simulink library "v2l"  (R2021b)
settings: Solver=VariableStepAuto  StartTime=0.0  StopTime=10.0  RelTol=1e-3
undefined symbols (not defined in the file or in its folder): KV2L_HVBattSOCLimit_pct, KV2L_SOCV2LSetLimit_pct
libraries: nmm x1, FVT_lib x1
settings Model: Creator=FVT23010  LastModifiedBy=FVT23010

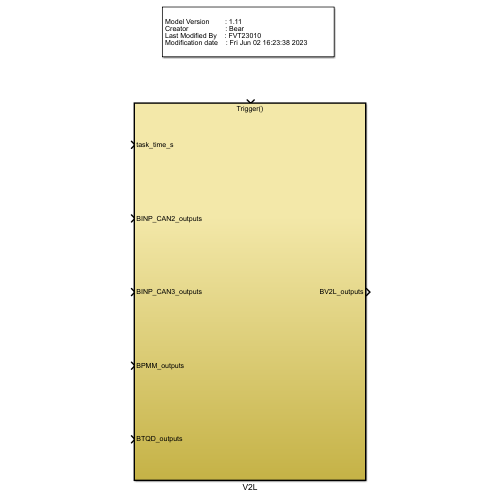
[thumbnail: Simulink's stored preview of the top-level diagram]
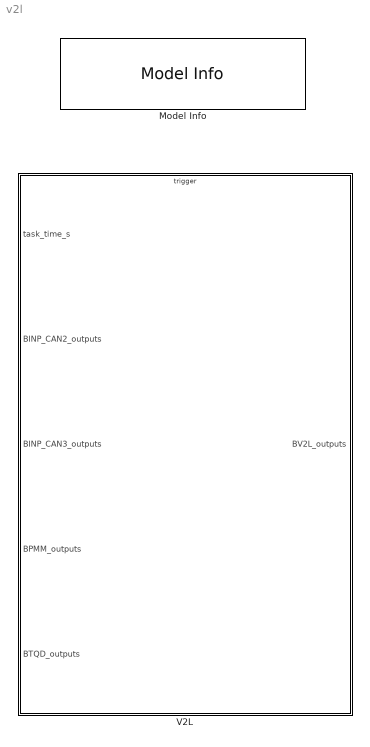
== system v2l ==
  Model Info : nmm/Model Info  InitialBlockCM=None  BlockCM=None  Frame=on  DisplayStringWithTags=|  HorizontalTextAlignment=Left  LeftAlignmentValue=0.02  SourceBlockDiagram=pmm  TagMaxNumber=20
      | Model Version        : %<ModelVersion>
      | Creator                   : Bear
      | Last Modified By    : %<LastModifiedBy>
      | Modification date    : %<LastModificationDate>
  V2L : Subsystem
      settings: RTWSystemCode=Nonreusable function  RTWFcnNameOpts=Use subsystem name  RTWFileNameOpts=Use subsystem name

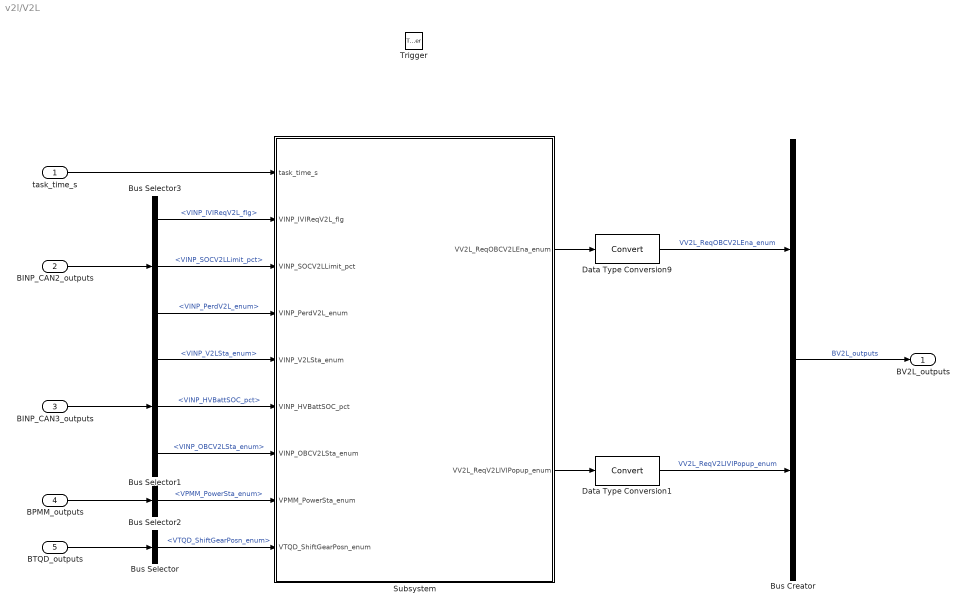
== system v2l/V2L ==
  task_time_s : Inport
  BINP_CAN2_outputs : Inport  Port=2  OutDataTypeStr=Bus: BINP_CAN2_outputs
  BINP_CAN3_outputs : Inport  Port=3  OutDataTypeStr=Bus: BINP_CAN3_outputs
  BPMM_outputs : Inport  Port=4  OutDataTypeStr=Bus: BPMM_outputs
  BTQD_outputs : Inport  Port=5  OutDataTypeStr=Bus: BTQD_outputs
  Trigger : TriggerPort  TriggerType=function-call  VariantControl=(inherit)  PortDimensions=1
  Bus Creator : BusCreator  Inputs=2  OutDataTypeStr=Bus: BV2L_outputs
  Bus Selector : BusSelector  OutputSignals=VTQD_ShiftGearPosn_enum
  Bus Selector1 : BusSelector  OutputSignals=VINP_V2LSta_enum,VINP_HVBattSOC_pct,VINP_OBCV2LSta_enum
  Bus Selector2 : BusSelector  OutputSignals=VPMM_PowerSta_enum
  Bus Selector3 : BusSelector  OutputSignals=VINP_IVIReqV2L_flg,VINP_SOCV2LLimit_pct,VINP_PerdV2L_enum
  Data Type Conversion1 : DataTypeConversion
  Data Type Conversion9 : DataTypeConversion
  Subsystem : Subsystem
  BV2L_outputs : Outport  OutDataTypeStr=Bus: BV2L_outputs
  wires:
  Bus Creator/1 -> BV2L_outputs/1  "BV2L_outputs"
  Subsystem/1(VV2L_ReqOBCV2LEna_enum) -> Data Type Conversion9/1
  Subsystem/2(VV2L_ReqV2LIVIPopup_enum) -> Data Type Conversion1/1
  task_time_s/1 -> Subsystem/1(task_time_s)
  BTQD_outputs/1 -> Bus Selector/1
  Bus Selector/1 -> Subsystem/9(VTQD_ShiftGearPosn_enum)  "<VTQD_ShiftGearPosn_enum>"
  BINP_CAN3_outputs/1 -> Bus Selector1/1
  Bus Selector1/2 -> Subsystem/6(VINP_HVBattSOC_pct)  "<VINP_HVBattSOC_pct>"
  BPMM_outputs/1 -> Bus Selector2/1
  Bus Selector2/1 -> Subsystem/8(VPMM_PowerSta_enum)  "<VPMM_PowerSta_enum>"
  BINP_CAN2_outputs/1 -> Bus Selector3/1
  Bus Selector3/2 -> Subsystem/3(VINP_SOCV2LLimit_pct)  "<VINP_SOCV2LLimit_pct>"
  Bus Selector3/1 -> Subsystem/2(VINP_IVIReqV2L_flg)  "<VINP_IVIReqV2L_flg>"
  Bus Selector3/3 -> Subsystem/4(VINP_PerdV2L_enum)  "<VINP_PerdV2L_enum>"
  Bus Selector1/1 -> Subsystem/5(VINP_V2LSta_enum)  "<VINP_V2LSta_enum>"
  Bus Selector1/3 -> Subsystem/7(VINP_OBCV2LSta_enum)  "<VINP_OBCV2LSta_enum>"
  Data Type Conversion9/1 -> Bus Creator/1  "VV2L_ReqOBCV2LEna_enum"
  Data Type Conversion1/1 -> Bus Creator/2  "VV2L_ReqV2LIVIPopup_enum"

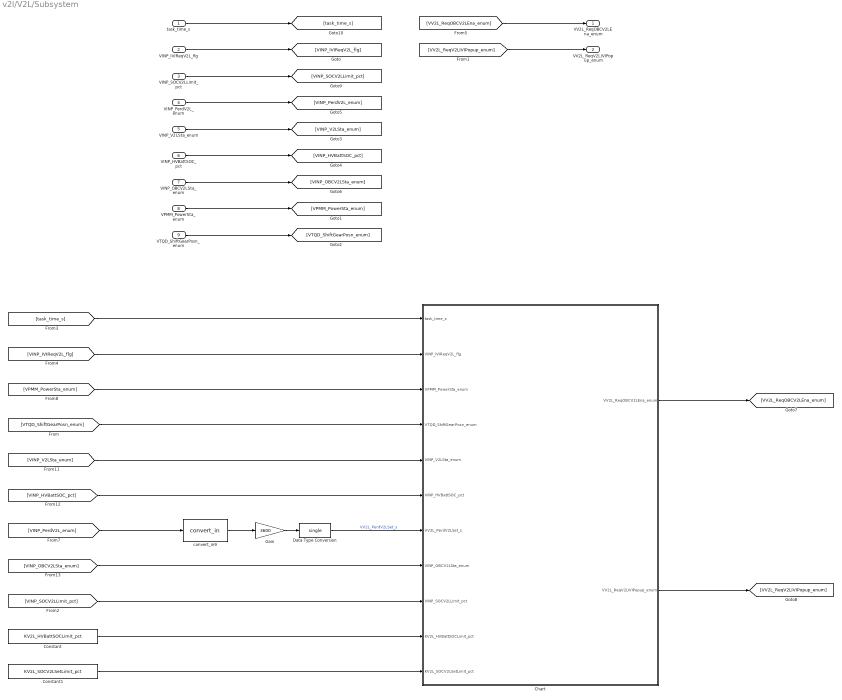
== system v2l/V2L/Subsystem ==
  task_time_s : Inport
  VINP_IVIReqV2L_flg : Inport  Port=2
  VINP_SOCV2LLimit_pct : Inport  Port=3
  VINP_PerdV2L_enum : Inport  Port=4
  VINP_V2LSta_enum : Inport  Port=5
  VINP_HVBattSOC_pct : Inport  Port=6
  VINP_OBCV2LSta_enum : Inport  Port=7
  VPMM_PowerSta_enum : Inport  Port=8
  VTQD_ShiftGearPosn_enum : Inport  Port=9
  Chart : Stateflow chart  TreatAsAtomicUnit=on
  Constant : Constant  Value=KV2L_HVBattSOCLimit_pct
  Constant1 : Constant  Value=KV2L_SOCV2LSetLimit_pct
  Data Type Conversion : DataTypeConversion  OutDataTypeStr=single
  Gain : Gain  Gain=3600
  convert_in9 : FVT_lib/hal/convert_in  gain=0.5  offset=0.5
  VV2L_ReqOBCV2LEna_enum : Outport
  VV2L_ReqV2LIVIPopup_enum : Outport  Port=2
  wires:
  task_time_s/1 -> [task_time_s]
  [VV2L_ReqOBCV2LEna_enum] -> VV2L_ReqOBCV2LEna_enum/1
  [task_time_s] -> Chart/1(task_time_s)
  Constant1/1 -> Chart/11(KV2L_SOCV2LSetLimit_pct)
  Chart/1(VV2L_ReqOBCV2LEna_enum) -> [VV2L_ReqOBCV2LEna_enum]
  VTQD_ShiftGearPosn_enum/1 -> [VTQD_ShiftGearPosn_enum]
  VINP_IVIReqV2L_flg/1 -> [VINP_IVIReqV2L_flg]
  VINP_SOCV2LLimit_pct/1 -> [VINP_SOCV2LLimit_pct]
  VINP_V2LSta_enum/1 -> [VINP_V2LSta_enum]
  VINP_OBCV2LSta_enum/1 -> [VINP_OBCV2LSta_enum]
  [VINP_HVBattSOC_pct] -> Chart/6(VINP_HVBattSOC_pct)
  Chart/2(VV2L_ReqV2LIVIPopup_enum) -> [VV2L_ReqV2LIVIPopup_enum]
  VINP_PerdV2L_enum/1 -> [VINP_PerdV2L_enum]
  [VINP_SOCV2LLimit_pct] -> Chart/9(VINP_SOCV2LLimit_pct)
  VPMM_PowerSta_enum/1 -> [VPMM_PowerSta_enum]
  [VINP_IVIReqV2L_flg] -> Chart/2(VINP_IVIReqV2L_flg)
  [VINP_V2LSta_enum] -> Chart/5(VINP_V2LSta_enum)
  [VINP_OBCV2LSta_enum] -> Chart/8(VINP_OBCV2LSta_enum)
  VINP_HVBattSOC_pct/1 -> [VINP_HVBattSOC_pct]
  [VPMM_PowerSta_enum] -> Chart/3(VPMM_PowerSta_enum)
  Constant/1 -> Chart/10(KV2L_HVBattSOCLimit_pct)
  [VV2L_ReqV2LIVIPopup_enum] -> VV2L_ReqV2LIVIPopup_enum/1
  [VTQD_ShiftGearPosn_enum] -> Chart/4(VTQD_ShiftGearPosn_enum)
  Data Type Conversion/1 -> Chart/7(VV2L_PerdV2LSet_s)  "VV2L_PerdV2LSet_s"
  Gain/1 -> Data Type Conversion/1
  [VINP_PerdV2L_enum] -> convert_in9/1
  convert_in9/1 -> Gain/1

== stateflow chart v2l/V2L/Subsystem/Chart ==
  state V2L
    en:
    VV2L_PerdV2LTimer_s = 0;
    VV2L_ReqOBCV2LEna_enum = ENUM_REQOBCV2L_NOREQUEST;
    VV2L_ReqV2LIVIPopup_enum = ENUM_REQV2LIVI_NOREQUEST;
    % 第一版先不考慮V2L放電模式下，更改設定時間的可能
    (default) -> (junction 102)
    V2L -> (junction 102) : {VV2L_ReqV2LIVIPopup_enum = ENUM_REQV2LIVI_NOREQUEST}
    (junction 102) -> (junction 16) [order 1] : [VINP_IVIReqV2L_flg]
    (junction 16) -> (junction 191) [order 1] : [VINP_HVBattSOC_pct > KV2L_HVBattSOCLimit_pct]
    (junction 191) -> (junction 45) [order 1] : [VINP_SOCV2LLimit_pct >= KV2L_SOCV2LSetLimit_pct]
    (junction 45) -> (junction 53) [order 1] : [VINP_HVBattSOC_pct > VINP_SOCV2LLimit_pct]
    (junction 53) -> (junction 168) [order 1] : [VV2L_PerdV2LSet_s > VV2L_PerdV2LTimer_s]
        | {VV2L_PerdV2LTimer_s += task_time_s;}
    (junction 168) -> (junction 217) [order 1] : [VTQD_ShiftGearPosn_enum == ENUM_GEARPOSNTOCAN_P && VPMM_PowerSta_enum == ENUM_POWERSTA_ON]
    (junction 217) -> (junction 180) [order 1] : [VINP_V2LSta_enum == ENUM_V2LSTA_PLUGIN || VINP_V2LSta_enum == ENUM_V2LSTA_SWON]
    (junction 180) -> (junction 59) [order 1] : [VINP_V2LSta_enum == ENUM_V2LSTA_SWON]
        | {VV2L_ReqOBCV2LEna_enum = ENUM_REQOBCV2L_EXTERNALDISCHRG;}
    (junction 59) -> (junction 61) [order 1] : [VINP_OBCV2LSta_enum == ENUM_OBCV2LSTA_FAULT]
    (junction 102) -> (junction 108) [order 2]
    (junction 16) -> (junction 200) [order 2] : {VV2L_ReqV2LIVIPopup_enum = ENUM_REQV2LIVI_SOCTOOLOW;}
    (junction 191) -> (junction 192) [order 2]
    (junction 45) -> (junction 203) [order 2] : {VV2L_ReqV2LIVIPopup_enum = ENUM_REQV2LIVI_STOPBYSOC;}
    (junction 53) -> (junction 205) [order 2] : {VV2L_ReqV2LIVIPopup_enum = ENUM_REQV2LIVI_TIMEUP;}
    (junction 168) -> (junction 173) [order 2]
    (junction 217) -> (junction 223) [order 2]
    (junction 180) -> (junction 226) [order 2] : {VV2L_ReqV2LIVIPopup_enum = ENUM_REQV2LIVI_PLUGINSWOFF;
        | VV2L_ReqOBCV2LEna_enum = ENUM_REQOBCV2L_NOREQUEST;
        | VV2L_PerdV2LTimer_s = 0;}
    (junction 59) -> (junction 218) [order 2]
    (junction 61) -> (junction 63) : {VV2L_ReqV2LIVIPopup_enum = ENUM_REQV2LIVI_FAULT;}
    (junction 173) -> (junction 167) [order 1] : [VINP_V2LSta_enum == ENUM_V2LSTA_NOPLUG]
    (junction 167) -> (junction 172)
    (junction 173) -> (junction 207) [order 2] : {VV2L_ReqV2LIVIPopup_enum = ENUM_REQV2LIVI_CHECKPLUG;}
    (junction 108) -> (junction 200)
    (junction 200) -> (junction 192)
    (junction 192) -> (junction 203)
    (junction 203) -> (junction 205)
    (junction 205) -> (junction 207)
    (junction 207) -> (junction 172)
    (junction 172) -> (junction 223)
    (junction 223) -> (junction 63)
    (junction 63) -> (junction 196) : {VV2L_ReqOBCV2LEna_enum = ENUM_REQOBCV2L_NOREQUEST;
        | VV2L_PerdV2LTimer_s = 0;}
  (default) -> V2L
  data: task_time_s input; VINP_IVIReqV2L_flg input; VPMM_PowerSta_enum input; VTQD_ShiftGearPosn_enum input; VINP_V2LSta_enum input; VINP_HVBattSOC_pct input; VV2L_PerdV2LSet_s input; VV2L_ReqOBCV2LEna_enum output uint8; VV2L_ReqV2LIVIPopup_enum output uint8; ENUM_GEARPOSNTOCAN_P parameter; ENUM_POWERSTA_ON parameter; ENUM_REQV2LIVI_CHECKPLUG parameter; ENUM_V2LSTA_NOPLUG parameter; ENUM_V2LSTA_PLUGIN parameter; ENUM_V2LSTA_SWON parameter; ENUM_REQV2LIVI_SOCTOOLOW parameter; ENUM_REQV2LIVI_FAULT parameter; ENUM_REQV2LIVI_TIMEUP parameter; ENUM_REQV2LIVI_PLUGINSWOFF parameter; VINP_OBCV2LSta_enum input; VV2L_PerdV2LTimer_s local double; ENUM_OBCV2LSTA_FAULT parameter; VINP_SOCV2LLimit_pct input; ENUM_REQV2LIVI_NOREQUEST parameter; ENUM_REQV2LIVI_STOPBYSOC parameter; KV2L_HVBattSOCLimit_pct input; KV2L_SOCV2LSetLimit_pct input; ENUM_REQOBCV2L_EXTERNALDISCHRG parameter; ENUM_REQOBCV2L_NOREQUEST parameter
